simulink library "DELAYS"  (R2019a)
settings: Solver=VariableStepAuto  StartTime=0.0  StopTime=10.0  RelTol=1e-3
libraries: xbsIndex_r4 x2
settings Model: Creator=mybur  LastModifiedBy=mybur

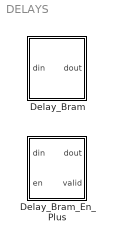
== system DELAYS ==
  Delay_Bram : Subsystem  mask{delay=3, bram_latency=1, bram_primitive="block", use_dsp=off, is_async=off}
      mask prompts: delay "Delay By:"; bram_latency "Bram Latency"; bram_primitive "Bram Primitive"; use_dsp "Use DSP48"; is_async "Asynchronous operation"
      mask init:
      | Simulink.Block.eval([gcb, '/delay_bram']);
      | 
      | delay_bram_subsys2bb_knit();
      mask TypeOptions bram_primitive: "block" | "auto" | "ultra" | "distributed"
      mask DialogControl Desc Prompt: A delay block that uses BRAM for its storage.
  Delay_Bram_En_Plus : Subsystem  mask{delay=2, bram_latency=2, bram_primitive="block"}
      mask prompts: delay "Enabled Delays"; bram_latency "Extra (unenabled) delay for BRAM Latency"; bram_primitive "Bram primitive"
      mask init:
      | Simulink.Block.eval([gcb, '/delay_bram_en_plus']);
      mask TypeOptions bram_primitive: "block" | "distributed" | "ultra" | "auto"
      mask DialogControl DescTextVar Prompt: A delay block that uses BRAM for its storage and only shifts when enabled. However, BRAM latency cannot be enabled, so output appears bram_latency clocks after an enable.

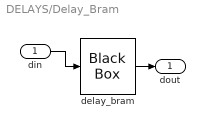
== system DELAYS/Delay_Bram ==
  din : Inport
  delay_bram : xbsIndex_r4/Black Box  init_code=delay_bram_config  sim_method=ISE Simulator  verbose=off  block_type=blackbox2
  dout : Outport
  wires:
  din/1 -> delay_bram/1
  delay_bram/1 -> dout/1

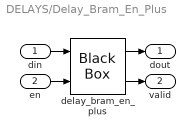
== system DELAYS/Delay_Bram_En_Plus ==
  din : Inport
  en : Inport  Port=2
  delay_bram_en_plus : xbsIndex_r4/Black Box  init_code=delay_bram_en_plus_config  sim_method=ISE Simulator  verbose=off  block_type=blackbox2
  dout : Outport
  valid : Outport  Port=2
  wires:
  delay_bram_en_plus/2 -> valid/1
  delay_bram_en_plus/1 -> dout/1
  din/1 -> delay_bram_en_plus/1
  en/1 -> delay_bram_en_plus/2
